simulink model "test"  (R2020b)
settings: Solver=VariableStepAuto  StartTime=0.0  StopTime=10.0  RelTol=1e-3
values from neighbouring files (symbols this model uses):
  sys_mimo = ss(A,B,C,0)    [SS_MIMO.m]
settings Model: Creator=krist  LastModifiedBy=krist

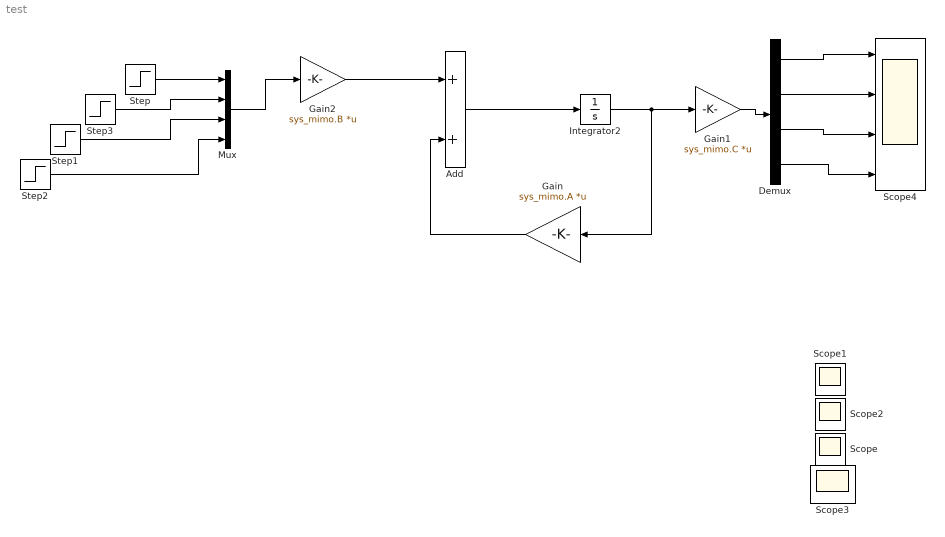
== system test ==
  Add : Sum
  Demux : Demux
  Gain : Gain  Gain=sys_mimo.A  Multiplication=Matrix(K*u)
  Gain1 : Gain  Gain=sys_mimo.C  Multiplication=Matrix(K*u)
  Gain2 : Gain  Gain=sys_mimo.B  Multiplication=Matrix(K*u)
  Integrator2 : Integrator
  Mux : Mux
  Scope{,1..3} (4 alike) : Scope
  Scope4 : Scope  NumInputPorts=4
  Step{,1..3} (4 alike) : Step  SampleTime=0
  wires:
  Integrator2/1 -> Gain/1, Gain1/1
  Add/1 -> Integrator2/1
  Gain/1 -> Add/2
  Gain2/1 -> Add/1
  Gain1/1 -> Demux/1
  Step/1 -> Mux/1
  Step3/1 -> Mux/2
  Step1/1 -> Mux/3
  Step2/1 -> Mux/4
  Mux/1 -> Gain2/1
  ? -> Scope1/1
  ? -> Scope2/1
  ? -> Scope/1
  ? -> Scope3/1
  Demux/1 -> Scope4/1
  Demux/2 -> Scope4/2
  Demux/3 -> Scope4/3
  Demux/4 -> Scope4/4
